simulink model "PID_Controller"  (R2025a)
settings: Solver=VariableStepAuto  StartTime=0.0  StopTime=10.0  RelTol=1e-3
settings Model: Creator=xing2  LastModifiedBy=xing2

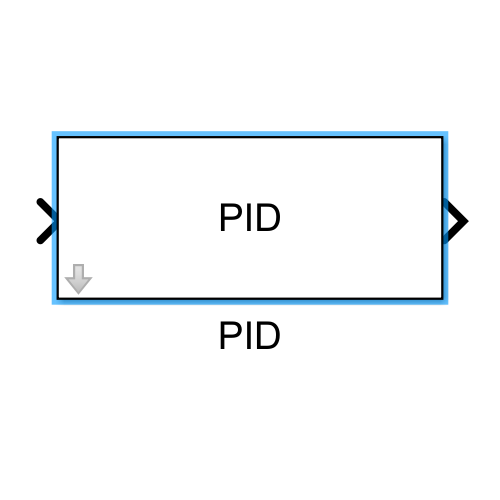
[thumbnail: Simulink's stored preview of the top-level diagram]
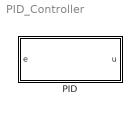
== system PID_Controller ==
  PID : Subsystem  mask{Kp=3, Ki=0.5, Kd=0.2, N=100, UL=10, LL=-10, Kaw=1}
      mask prompts: UL "Upper Limit"; LL "Lower Limit"; Kaw "Anti-Windup Gain"
      mask help: PID Controller with anti-windup and derivative filtering
      mask Display: disp('PID');

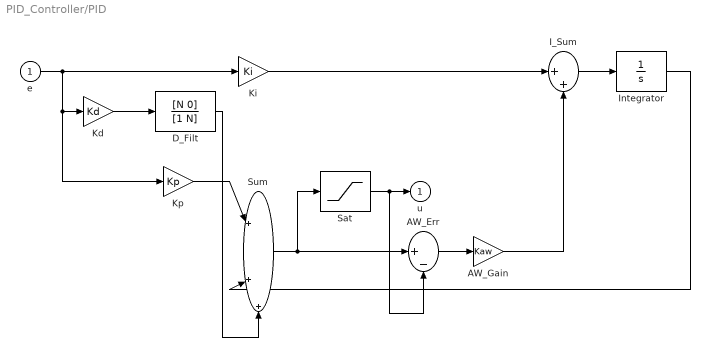
== system PID_Controller/PID ==
  e : Inport
  AW_Err : Sum  Inputs=|+-
  AW_Gain : Gain  Gain=Kaw
  D_Filt : TransferFcn  Numerator=[N 0]  Denominator=[1 N]
  I_Sum : Sum  Inputs=|++
  Integrator : Integrator
  Kd : Gain  Gain=Kd
  Ki : Gain  Gain=Ki
  Kp : Gain  Gain=Kp
  Sat : Saturate  UpperLimit=UL  LowerLimit=LL
  Sum : Sum  Inputs=|+++
  u : Outport
  wires:
  e/1 -> Kp/1, Kd/1, Ki/1
  AW_Gain/1 -> I_Sum/2
  Kd/1 -> D_Filt/1
  Sat/1 -> AW_Err/2, u/1
  Sum/1 -> AW_Err/1, Sat/1
  Ki/1 -> I_Sum/1
  Kp/1 -> Sum/1
  D_Filt/1 -> Sum/3
  AW_Err/1 -> AW_Gain/1
  I_Sum/1 -> Integrator/1
  Integrator/1 -> Sum/2
